simulink model "Anna_final"  (R2017b)
settings: Solver=ode45  StartTime=0.0  StopTime=1  RelTol=1e-3  EnableMultiTasking=on
undefined symbols (not defined in the file): Acid, Lead
libraries: powerlib x32, simulink x4, powerlib_extras x3, electricdrivelib x1
settings Model: Creator=Vipin  LastModifiedBy=tijubaby
settings DataIOCC: LimitDataPoints=on  SaveFormat=Array  SignalLoggingSaveFormat=ModelDataLogs
settings OptimizationCC: ExpressionDepthLimit=2147483647  LifeSpan=inf
settings DebuggingCC: UnderspecifiedInitializationDetection=Classic  MergeDetectMultiDrivingBlocksExec=none  SolverPrmCheckMsg=warning  MultiTaskDSMMsg=warning  MultiTaskCondExecSysMsg=none  FcnCallInpInsideContextMsg=warning  StateNameClashWarn=warning  StrictBusMsg=None  SFUnexpectedBacktrackingDiag=warning  SFNoUnconditionalDefaultTransitionDiag=warning  SFExecutionAtInitializationDiag=none
settings HardwareCC: ProdBitPerPointer=32  ProdBitPerSizeT=32  ProdBitPerPtrDiffT=32  ProdLargestAtomicFloat=None  ProdIntDivRoundTo=Undefined  ProdEndianess=Unspecified  ProdWordSize=32  ProdHWDeviceType=32-bit Generic
settings ModelReferenceCC: PropagateSignalLabelsOutOfModel=off
settings CodeAppCC: StateflowObjectComments=on
settings GRTTargetCC: TargetLangStandard=C89/C90 (ANSI)  GeneratePreprocessorConditionals=Disable all  CombineOutputUpdateFcns=off  GRTInterface=on
settings ConfigComp: CovMetricSettings=dw  CovHtmlReporting=on  CovSaveCumulativeToWorkspaceVar=on  CovSaveSingleToWorkspaceVar=on  CovExternalEMLEnable=off
settings SimscapeCC: SimscapeNormalizeSystem=off

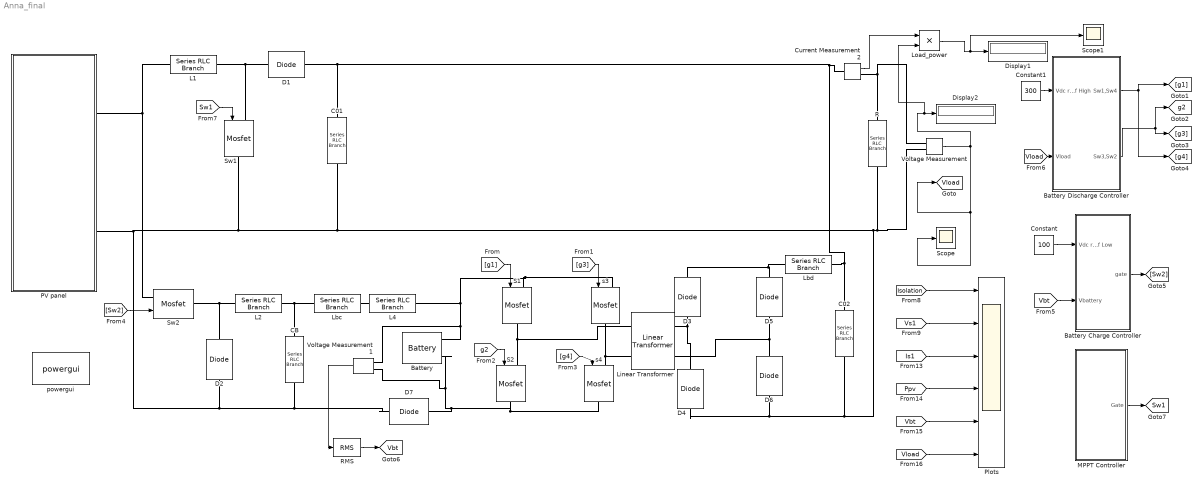
== system Anna_final ==
  Battery : electricdrivelib/Extra Sources/Battery  BatType=Lead-Acid  ShowTempParam=off  ThermalPreset=no  ShowAgeParam=off  NomV=100  NomQ=1  SOC=100  Batt_Tr=30  PresetModel=on  MaxQ=1.0417  MinV=75  FullV=108.8816  Dis_rate=0.2  R=1  Normal_OP=0.31028  expZone="[101.8092   0.003333333]"  current=[6.5 13 32.5]  Units=Ampere-hour  Tci=20  NomT=20  T2=-30  MaxQ2=4.8  FullV2=7.1  Normal_OP2=5.655  expZone2="[6.58           1]"  Rca=0.6  ti=2000  Dp=0  Neq0=0  Tsim=1e6  Ta1=25  Qeol=5.4*0.9  Reol=0.013333*1.2  Char_age=[2.3478, 3]  Dis_age=[2.3478, 10]  N1=1500  N2=10500  N3=1000  N4=1400  Ta2=45  N5=950
  Battery Charge Controller : Subsystem
  Battery Discharge Controller : Subsystem
  C01 : powerlib/Elements/Series RLC Branch  LConnTagsString=__new0  RConnTagsString=__new0  BranchType=C  Resistance=1  Inductance=1e-3  SetiL0=off  InitialCurrent=0  Capacitance=100e-6  Setx0=off  InitialVoltage=0  Measurements=Branch current
  C02 : powerlib/Elements/Series RLC Branch  LConnTagsString=__new0  RConnTagsString=__new0  BranchType=C  Resistance=1  Inductance=1e-3  SetiL0=off  InitialCurrent=0  Capacitance=100e-6  Setx0=off  InitialVoltage=0  Measurements=Branch current
  CB : powerlib/Elements/Series RLC Branch  LConnTagsString=__new0  RConnTagsString=__new0  BranchType=C  Resistance=1  Inductance=1e-3  SetiL0=off  InitialCurrent=0  Capacitance=100e-6  Setx0=off  InitialVoltage=0  Measurements=Branch current
  Constant : Constant  Value=100
  Constant1 : Constant  Value=300
  Current Measurement2 : powerlib/Measurements/Current Measurement  PhasorSimulation=off  OutputType=Complex  PSBequivalent=0
  D{1..6} (6 alike) : powerlib/Power Electronics/Diode  Ron=0.001  Lon=0  Vf=0.8  IC=0  UseSnubber=off  Rs=500  Cs=250e-9  Measurements=off
  D7 : powerlib/Power Electronics/Diode  Ron=0.00001  Lon=0  Vf=0.8  IC=0  UseSnubber=off  Rs=500  Cs=250e-9  Measurements=off
  Display1 : Display
      settings: Decimation=2000
  Display2 : Display
      settings: Decimation=2000
  L1 : powerlib/Elements/Series RLC Branch  LConnTagsString=__new0  RConnTagsString=__new0  BranchType=L  Resistance=1  Inductance=1.5e-3  SetiL0=off  InitialCurrent=0  Capacitance=1e-6  Setx0=off  InitialVoltage=0  Measurements=Branch current
  L2 : powerlib/Elements/Series RLC Branch  LConnTagsString=__new0  RConnTagsString=__new0  BranchType=L  Resistance=1  Inductance=1e-3  SetiL0=off  InitialCurrent=0  Capacitance=1e-6  Setx0=off  InitialVoltage=0  Measurements=Branch current
  L4 : powerlib/Elements/Series RLC Branch  LConnTagsString=__new0  RConnTagsString=__new0  BranchType=R  Resistance=1  Inductance=1e-3  SetiL0=off  InitialCurrent=0  Capacitance=1e-6  Setx0=off  InitialVoltage=0  Measurements=Branch current
  Lbc : powerlib/Elements/Series RLC Branch  LConnTagsString=__new0  RConnTagsString=__new0  BranchType=L  Resistance=1  Inductance=10e-6  SetiL0=off  InitialCurrent=0  Capacitance=1e-6  Setx0=off  InitialVoltage=0  Measurements=Branch current
  Lbd : powerlib/Elements/Series RLC Branch  LConnTagsString=__new0  RConnTagsString=__new0  BranchType=L  Resistance=1  Inductance=2e-3  SetiL0=off  InitialCurrent=0  Capacitance=1e-6  Setx0=off  InitialVoltage=0  Measurements=Branch current
  Linear Transformer : powerlib/Elements/Linear Transformer  UNITS=SI  NominalPower=[1000 40e3 ]  winding1=[20 0.008 3e-07]  winding2=[160 0.072 2.7e-06]  ThreeWindings=off  winding3=[3.15e+05 0.7938 0.084225]  RmLm=[2000 0.0001487]  Measurements=None  DataType=on
  Load_power : Product  RndMeth=Zero
  MPPT Controller : Subsystem
  PV panel : Subsystem
  Plots : Scope  NumInputPorts=6
  R : powerlib/Elements/Series RLC Branch  LConnTagsString=__new0  RConnTagsString=__new0  BranchType=R  Resistance=800  Inductance=1e-3  SetiL0=off  InitialCurrent=0  Capacitance=1e-6  Setx0=off  InitialVoltage=0  Measurements=None
  RMS : powerlib_extras/Measurements/RMS  f1=50
  S1 : powerlib/Power Electronics/Mosfet  Ron=0.1  Lon=0  Rd=0.01  Vfd=0  IC=0  Rs=1e5  Cs=inf  Measurements=off
  S2 : powerlib/Power Electronics/Mosfet  Ron=0.1  Lon=0  Rd=0.01  Vfd=0  IC=0  Rs=1e5  Cs=inf  Measurements=off
  Scope : Scope
  Scope1 : Scope
  Sw1 : powerlib/Power Electronics/Mosfet  Ron=0.1  Lon=0  Rd=0.01  Vfd=0  IC=0  Rs=1e5  Cs=inf  Measurements=off
  Sw2 : powerlib/Power Electronics/Mosfet  Ron=0.1  Lon=0  Rd=0.01  Vfd=0  IC=0  Rs=1e5  Cs=inf  Measurements=off
  Voltage Measurement : powerlib/Measurements/Voltage Measurement  PhasorSimulation=off  OutputType=Complex  PSBequivalent=0
  Voltage Measurement1 : powerlib/Measurements/Voltage Measurement  PhasorSimulation=off  OutputType=Complex  PSBequivalent=0
  powergui : powerlib/powergui  Priority=1  SimulationMode=Discrete  SampleTime=1e-6  frequency=60  Iterations=50  frequencyindice=0  Pbase=100e6  ErrMax=1e-4  UnitsV=kV  UnitsW=MW  buscounter=0  FunctionMessages=off  echomessages=off  EnableUseOfTLC=off  CurrentSourceSwitches=off  DisableSnubberDevices=off  DisableRonSwitches=off  DisableVfSwitches=off  DisplayEquations=off  SolverType=Tustin  Interpol=off  ExternalGateDelay=off  methode=off  Ts=0  x0status=blocks  SPID=off  SwTol=0  HookPort=off  RestoreLinks=warning  ResistiveCurrentMeasurement=off  Frange=[0:2:500]  Ylog=off  Xlog=on  ShowGrid=off  save=off  variable=ZData  structure=0  ZoomFFT=off  StartTime=0.0  cycles=1  DisplayStyle=1  fundamental=60  FreqAxis=off  MaxFrequency=1000  frequencyindicesteady=1  RmsSteady=1  display=off
  s3 : powerlib/Power Electronics/Mosfet  Ron=0.1  Lon=0  Rd=0.01  Vfd=0  IC=0  Rs=1e5  Cs=inf  Measurements=off
  s4 : powerlib/Power Electronics/Mosfet  Ron=0.1  Lon=0  Rd=0.01  Vfd=0  IC=0  Rs=1e5  Cs=inf  Measurements=off
  tag scope: Sw1=global, Vbt=global, Vload=global, g2=global
  wires:
  MPPT Controller/1(Gate) -> [Sw1]
  Battery Charge Controller/1(gate) -> [Sw2]
  Voltage Measurement/1 -> [Vload], Scope/1, Load_power/2, Display2/1
  RMS/1 -> [Vbt]
  Constant/1 -> Battery Charge Controller/1(Vdc ref Low)
  [g1] -> S1/1
  [g3] -> s3/1
  [g4] -> s4/1
  [g2] -> S2/1
  Battery Discharge Controller/2(Sw3,Sw2) -> [g3], [g2]
  Constant1/1 -> Battery Discharge Controller/1(Vdc ref High)
  Battery Discharge Controller/1(Sw1,Sw4) -> [g4], [g1]
  [Vload] -> Battery Discharge Controller/2(Vload)
  Voltage Measurement1/1 -> RMS/1
  [Sw2] -> Sw2/1
  [Vbt] -> Battery Charge Controller/2(Vbattery)
  [Sw1] -> Sw1/1
  [Is1] -> Plots/3
  [Vload] -> Plots/6
  [Vbt] -> Plots/5
  [Ppv] -> Plots/4
  [Vs1] -> Plots/2
  [Isolation] -> Plots/1
  Current Measurement2/1 -> Load_power/1
  Load_power/1 -> Scope1/1, Display1/1
  connections:
  L1/RConn1 -- Sw1/LConn1 -- D1/LConn1
  L1/LConn1 -- Sw2/LConn1 -- PV panel/LConn1
  Voltage Measurement/LConn1 -- Current Measurement2/RConn1 -- R/LConn1
  Sw2/RConn1 -- D2/RConn1 -- L2/LConn1
  L2/RConn1 -- Lbc/LConn1 -- CB/LConn1
  Lbc/RConn1 -- L4/LConn1
  S1/LConn1 -- Battery/LConn1 -- Voltage Measurement1/LConn1 -- L4/RConn1 -- s3/LConn1
  S2/LConn1 -- Linear Transformer/LConn1 -- S1/RConn1
  s4/LConn1 -- Linear Transformer/LConn2 -- s3/RConn1
  D4/RConn1 -- Linear Transformer/RConn1 -- D3/LConn1
  D6/RConn1 -- D5/LConn1 -- Linear Transformer/RConn2
  D3/RConn1 -- Lbd/LConn1 -- D5/RConn1
  Sw1/RConn1 -- D6/LConn1 -- D4/LConn1 -- C02/RConn1 -- Voltage Measurement/LConn2 -- R/RConn1 -- C01/RConn1 -- D2/LConn1 -- D7/RConn1 -- CB/RConn1 -- PV panel/LConn2
  S2/RConn1 -- Battery/LConn2 -- Voltage Measurement1/LConn2 -- D7/LConn1 -- s4/RConn1
  Lbd/RConn1 -- Current Measurement2/LConn1 -- C01/LConn1 -- D1/RConn1 -- C02/LConn1

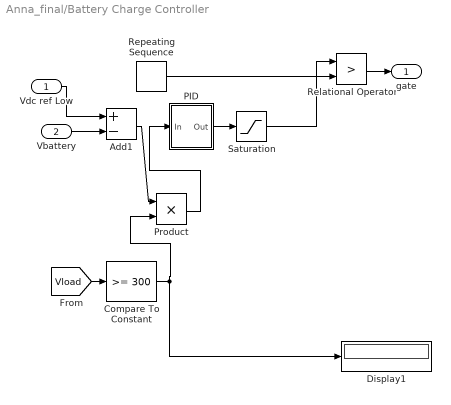
== system Anna_final/Battery Charge Controller ==
  Vdc ref Low : Inport
  Vbattery : Inport  Port=2
  Add1 : Sum  Inputs=+-
  Compare To Constant : simulink/Logic and Bit Operations/Compare To Constant  relop=>=  const=300  OutDataTypeStr=boolean
  Display1 : Display
      settings: Decimation=2000
  PID : Subsystem
  Product : Product
  Relational Operator : RelationalOperator  Operator=>  OutDataTypeStr=boolean  RndMeth=Nearest
  Repeating Sequence : simulink/Sources/Repeating Sequence  rep_seq_t=[0 50e-6]  rep_seq_y=[0 1]
  Saturation : Saturate  UpperLimit=1  LowerLimit=-1
  gate : Outport
  wires:
  Add1/1 -> Product/1
  PID/1(Out) -> Saturation/1
  Repeating Sequence/1 -> Relational Operator/2
  Saturation/1 -> Relational Operator/1
  Vbattery/1 -> Add1/2
  Relational Operator/1 -> gate/1
  Vdc ref Low/1 -> Add1/1
  Product/1 -> PID/1(In)
  Compare To Constant/1 -> Product/2, Display1/1
  [Vload] -> Compare To Constant/1

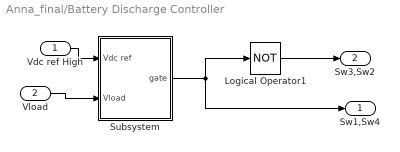
== system Anna_final/Battery Discharge Controller ==
  Vdc ref High : Inport
  Vload : Inport  Port=2
  Logical Operator1 : Logic  Operator=NOT  AllPortsSameDT=off  OutDataTypeStr=boolean
  Subsystem : Subsystem
  Sw1,Sw4 : Outport
  Sw3,Sw2 : Outport  Port=2
  wires:
  Vdc ref High/1 -> Subsystem/1(Vdc ref)
  Vload/1 -> Subsystem/2(Vload)
  Logical Operator1/1 -> Sw3,Sw2/1
  Subsystem/1(gate) -> Sw1,Sw4/1, Logical Operator1/1

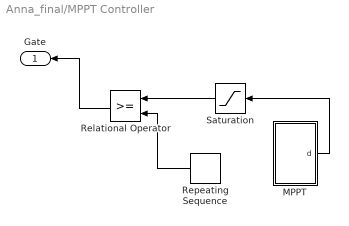
== system Anna_final/MPPT Controller ==
  MPPT : Subsystem
  Relational Operator : RelationalOperator  OutDataTypeStr=boolean  RndMeth=Nearest
  Repeating Sequence : simulink/Sources/Repeating Sequence  rep_seq_t=[0 50e-6]  rep_seq_y=[0 1]
  Saturation : Saturate  UpperLimit=0.75  LowerLimit=0.67
  Gate : Outport
  wires:
  Relational Operator/1 -> Gate/1
  Saturation/1 -> Relational Operator/1
  Repeating Sequence/1 -> Relational Operator/2
  MPPT/1(d) -> Saturation/1

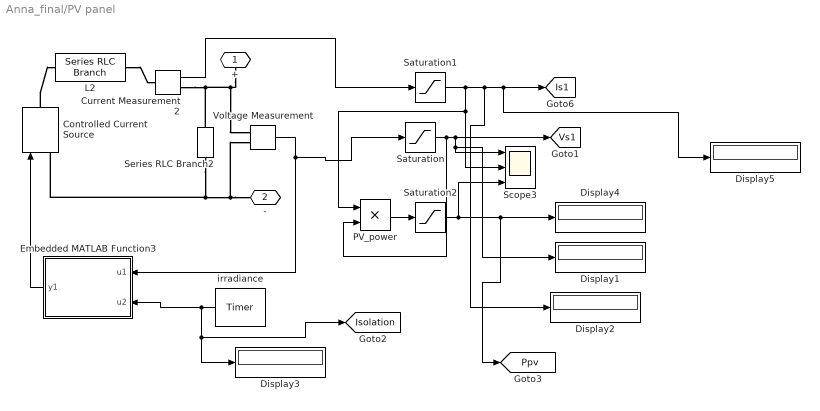
== system Anna_final/PV panel ==
  Controlled Current Source : powerlib/Electrical Sources/Controlled Current Source  Initialize=on  Source_Type=DC  Amplitude=0  Phase=0  Frequency=0  Measurements=None
  Current Measurement2 : powerlib/Measurements/Current Measurement  PhasorSimulation=off  OutputType=Complex  PSBequivalent=0
  Display{1..5} (5 alike) : Display
      settings: Decimation=2000
  Embedded MATLAB Function3 : MATLAB Function  TreatAsAtomicUnit=on
  L2 : powerlib/Elements/Series RLC Branch  LConnTagsString=__new0  RConnTagsString=__new0  BranchType=R  Resistance=1  Inductance=1e-3  SetiL0=off  InitialCurrent=0  Capacitance=1e-6  Setx0=off  InitialVoltage=0  Measurements=Branch current
  PV_power : Product  RndMeth=Zero
  Saturation : Saturate  UpperLimit=100  LowerLimit=0
  Saturation1 : Saturate  UpperLimit=10  LowerLimit=0
  Saturation2 : Saturate  UpperLimit=300  LowerLimit=0
  Scope3 : Scope  NumInputPorts=3
  Series RLC Branch2 : powerlib/Elements/Series RLC Branch  LConnTagsString=__new0  RConnTagsString=__new0  BranchType=C  Resistance=0  Inductance=1e-6  SetiL0=off  InitialCurrent=0  Capacitance=1e-3  Setx0=on  InitialVoltage=0  Measurements=None
  Voltage Measurement : powerlib/Measurements/Voltage Measurement  PhasorSimulation=off  OutputType=Complex  PSBequivalent=0
  irradiance : powerlib_extras/Control  Blocks/Timer  t=[0 .4 .5 .7 1]  e=[0 500 1000 500 0]
  + : PMIOPort  Port=1  Side=Left
  - : PMIOPort  Port=2  Side=Left
  tag scope: Is1=global, Isolation=global, Ppv=global, Vs1=global
  wires:
  Embedded MATLAB Function3/1(y1) -> Controlled Current Source/1
  Voltage Measurement/1 -> Embedded MATLAB Function3/1(u1), Saturation/1
  Current Measurement2/1 -> Saturation1/1
  irradiance/1 -> [Isolation], Display3/1, Embedded MATLAB Function3/2(u2)
  Saturation/1 -> PV_power/2, Display1/1, Scope3/1, [Vs1]
  PV_power/1 -> Saturation2/1
  Saturation2/1 -> [Ppv], Display4/1, Scope3/3
  Saturation1/1 -> Display2/1, Display5/1, [Is1], PV_power/1, Scope3/2
  connections:
  Current Measurement2/RConn1 -- +/RConn1 -- Voltage Measurement/LConn1 -- Series RLC Branch2/LConn1
  -/RConn1 -- Series RLC Branch2/RConn1 -- Controlled Current Source/LConn1 -- Voltage Measurement/LConn2
  L2/RConn1 -- Current Measurement2/LConn1
  Controlled Current Source/RConn1 -- L2/LConn1

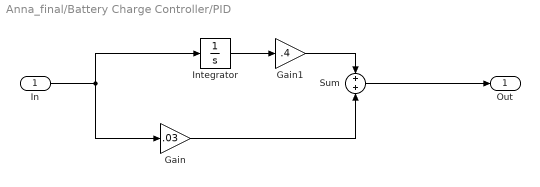
== system Anna_final/Battery Charge Controller/PID ==
  In : Inport
  Gain : Gain  Gain=.03
  Gain1 : Gain  Gain=.4
  Integrator : Integrator
  Sum : Sum  Inputs=+|+
  Out : Outport
  wires:
  Gain/1 -> Sum/2
  Gain1/1 -> Sum/1
  Sum/1 -> Out/1
  Integrator/1 -> Gain1/1
  In/1 -> Integrator/1, Gain/1

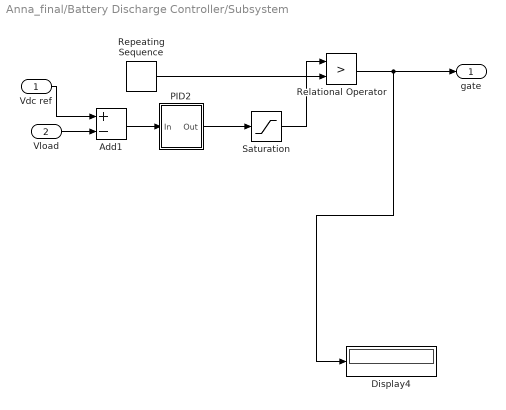
== system Anna_final/Battery Discharge Controller/Subsystem ==
  Vdc ref : Inport
  Vload : Inport  Port=2
  Add1 : Sum  Inputs=+-
  Display4 : Display
      settings: Decimation=2000
  PID2 : Subsystem
  Relational Operator : RelationalOperator  Operator=>  OutDataTypeStr=boolean  RndMeth=Nearest
  Repeating Sequence : simulink/Sources/Repeating Sequence  rep_seq_t=[0 50e-6]  rep_seq_y=[0 1]
  Saturation : Saturate  UpperLimit=.2  LowerLimit=0
  gate : Outport
  wires:
  PID2/1(Out) -> Saturation/1
  Repeating Sequence/1 -> Relational Operator/2
  Saturation/1 -> Relational Operator/1
  Vload/1 -> Add1/2
  Relational Operator/1 -> Display4/1, gate/1
  Vdc ref/1 -> Add1/1
  Add1/1 -> PID2/1(In)

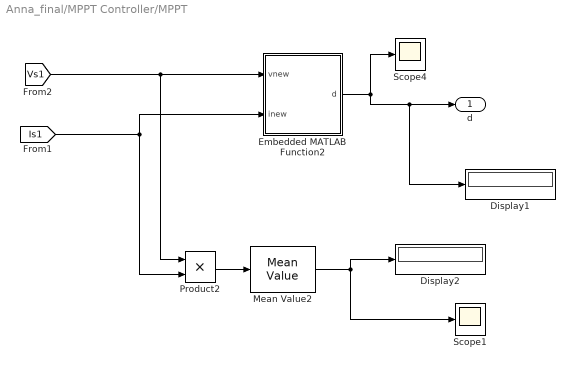
== system Anna_final/MPPT Controller/MPPT ==
  Display1 : Display
      settings: Decimation=2000
  Display2 : Display
      settings: Decimation=2000
  Embedded MATLAB Function2 : MATLAB Function  TreatAsAtomicUnit=on
  Mean Value2 : powerlib_extras/Measurements/Mean Value  Period=1/50
  Product2 : Product  RndMeth=Zero
  Scope1 : Scope
  Scope4 : Scope
  d : Outport
  wires:
  Mean Value2/1 -> Display2/1, Scope1/1
  Product2/1 -> Mean Value2/1
  [Is1] -> Product2/2, Embedded MATLAB Function2/2(inew)
  [Vs1] -> Product2/1, Embedded MATLAB Function2/1(vnew)
  Embedded MATLAB Function2/1(d) -> Display1/1, d/1, Scope4/1

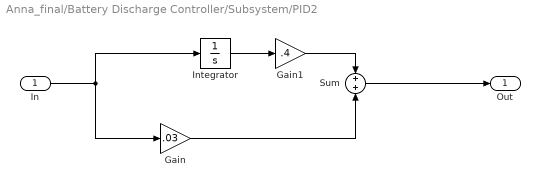
== system Anna_final/Battery Discharge Controller/Subsystem/PID2 ==
  In : Inport
  Gain : Gain  Gain=.03
  Gain1 : Gain  Gain=.4
  Integrator : Integrator
  Sum : Sum  Inputs=+|+
  Out : Outport
  wires:
  Gain/1 -> Sum/2
  Gain1/1 -> Sum/1
  Sum/1 -> Out/1
  Integrator/1 -> Gain1/1
  In/1 -> Integrator/1, Gain/1

== matlab function Anna_final/MPPT Controller/MPPT/Embedded MATLAB Function2 ==
  data: vnew input; inew input; d output
function d = fcn(vnew,inew)

dmax=0.9;
dmin=0.4;
dini=0.6;
deld=1e-4;
pnew=vnew*inew;
persistent pold dold vold c;

if isempty(pold)
    pold=0;
    vold=0;
    dold=dini;
    c=-50;
end
delp=pnew-pold;
delv=vnew-vold;
c=c+1;

if (c==50)
    if (delp>0)
       if (delv<0)
       d=dold+deld;
       else
       d=dold-deld;
       end
    else
       if (delv<0);
           d=dold-deld;
       else
           d=dold+deld;
       end 
    end
if (d>dmax || d<dmin)
    d=dold;
end
pold=pnew;
vold=vnew;
dold=d;
c=0;
else
    d=dold;
end
end

== matlab function Anna_final/PV panel/Embedded MATLAB Function3 ==
  data: u1 input; y1 output; u2 input
function y1 = fcn(u1,u2)
Rs = 0.01;%cell series resistance
Rp = 10000;% cell shunt resistance
Ipho = 2;
Iro  = 1000;
Ir   = u2;% irradiance
T    = 27;% Temperature
Np   = 17;% # of parallel connected cells
Ns   = 220;% # of series connected cells
Iph  = Ipho * Ir/Iro;
k    = 1.38e-23;% Boltzmann’s constant 
q    = 1.6e-19;% Electron charge
Vt   = k*(T+273)/q;
N1   = 1.5;% Diode ideality factor
TIPH1= 0;
Tmeas= 27;%measured temperature
Iph  = Iph * (1 + TIPH1*(T-Tmeas));
EG   = 1.11;% Band gap energy; 1.12eV (Si), 1.42 (GaAs)%   1.5 (CdTe), 1.75 (amorphous Si)
Is   = 1e-8;
TXIS1= 3;
TRS1 = 0;
TRP1 = 0;
i=1;
for y=1:10
   f = i*(1+Rs/Rp) - Np*Iph + (u1*Np*Ns)/Rp + Np*Is*(exp((u1/Ns+i*Rs/Np)/Vt)-1);
   fd=   (1+Rs/Rp) + Is*Rs/Vt*exp((u1/Ns+i*Rs/Np)/Vt);
   i = i - f/fd;
end
y1 = i;
end
